simulink model "Practico_Simulink"  (R2017a)
settings: Solver=VariableStepAuto  StartTime=0.0  StopTime=10.0  RelTol=1e-3
values from neighbouring files (symbols this model uses):
  ac = [(-r1-r2)/l1,-r1/l1,0;-r1/l2,(-r1-r3)/l2,1/l2;0,-1/c,-1/(r4*c)]    [CircuitoRLC.m]
  ad = Fds.A    [CircuitoRLC.m]
  bc = [1/l1;0;1/(r4*c)]    [CircuitoRLC.m]
  bd = Fds.B    [CircuitoRLC.m]
  cc = [0,0,-1]    [CircuitoRLC.m]
  cd = Fds.C    [CircuitoRLC.m]
  dc = 1    [CircuitoRLC.m]
  dd = Fds.D    [CircuitoRLC.m]
settings Model: Creator=franj  LastModifiedBy=franj

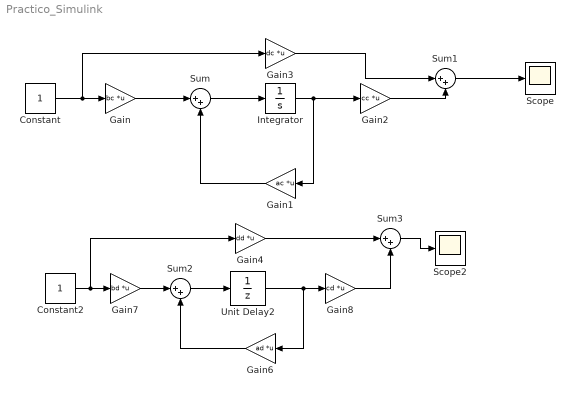
== system Practico_Simulink ==
  Constant : Constant
  Constant2 : Constant
  Gain : Gain  Gain=bc  Multiplication=Matrix(K*u)
  Gain1 : Gain  Gain=ac  Multiplication=Matrix(K*u)
  Gain2 : Gain  Gain=cc  Multiplication=Matrix(K*u)
  Gain3 : Gain  Gain=dc  Multiplication=Matrix(K*u)
  Gain4 : Gain  Gain=dd  Multiplication=Matrix(K*u)
  Gain6 : Gain  Gain=ad  Multiplication=Matrix(K*u)
  Gain7 : Gain  Gain=bd  Multiplication=Matrix(K*u)
  Gain8 : Gain  Gain=cd  Multiplication=Matrix(K*u)
  Integrator : Integrator
  Scope : Scope
  Scope2 : Scope
  Sum{,1..3} (4 alike) : Sum  Inputs=|++
  Unit Delay2 : UnitDelay  SampleTime=-1
  wires:
  Constant/1 -> Gain3/1, Gain/1
  Gain/1 -> Sum/1
  Sum/1 -> Integrator/1
  Gain1/1 -> Sum/2
  Integrator/1 -> Gain2/1, Gain1/1
  Gain2/1 -> Sum1/2
  Gain3/1 -> Sum1/1
  Sum1/1 -> Scope/1
  Sum2/1 -> Unit Delay2/1
  Constant2/1 -> Gain4/1, Gain7/1
  Gain7/1 -> Sum2/1
  Unit Delay2/1 -> Gain6/1, Gain8/1
  Gain6/1 -> Sum2/2
  Gain8/1 -> Sum3/2
  Gain4/1 -> Sum3/1
  Sum3/1 -> Scope2/1
